simulink model "lowPassFilter"  (R2023a)
settings: Solver=VariableStepAuto  StartTime=0.0  StopTime=10.0  RelTol=1e-3
settings Model: Creator=z'k'x  LastModifiedBy=z'k'x

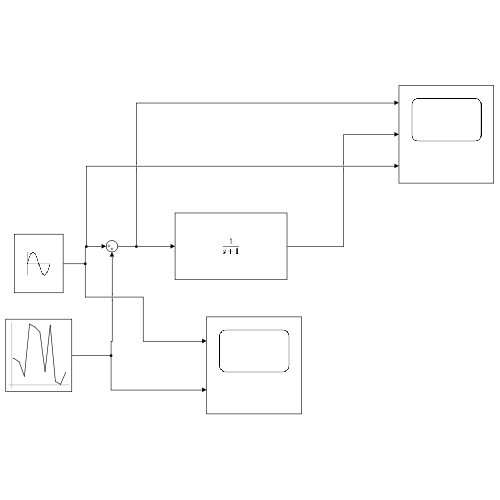
[thumbnail: Simulink's stored preview of the top-level diagram]
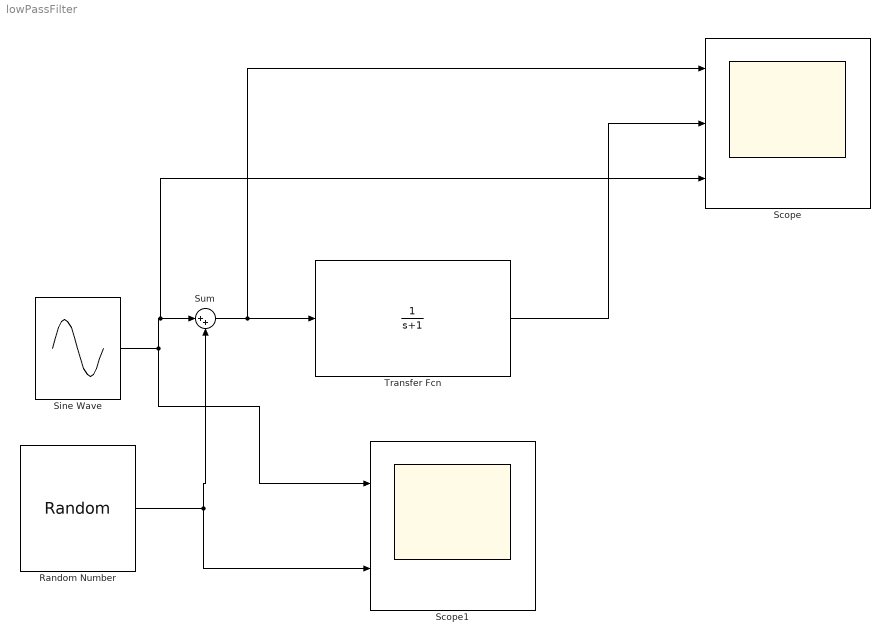
== system lowPassFilter ==
  Random Number : RandomNumber  Variance=0.1  SampleTime=0.01
  Scope : Scope  NumInputPorts=3
  Scope1 : Scope  NumInputPorts=2
  Sine Wave : Sin  SampleTime=0
  Sum : Sum  Inputs=|++
  Transfer Fcn : TransferFcn  Denominator=[1 1]
  wires:
  Sum/1 -> Scope/1, Transfer Fcn/1
  Sine Wave/1 -> Scope1/1, Scope/3, Sum/1
  Random Number/1 -> Scope1/2, Sum/2
  Transfer Fcn/1 -> Scope/2
